simulink model "Project"  (R2024a)
settings: Solver=FixedStepDiscrete  StartTime=0.0  StopTime=10.0  FixedStep=1e-3  RelTol=1e-3
settings Model: Creator=User  LastModifiedBy=User
settings OptimizationCC: DefaultParameterBehavior=Inlined  EnhancedBackFolding=on  PassReuseOutputArgsAs=Individual arguments  ZeroExternalMemoryAtStartup=off  ZeroInternalMemoryAtStartup=off  OptimizeBlockOrder=speed  DifferentSizesBufferReuse=on  OptimizationCustomize=off  EfficientTunableParamExpr=on
settings DebuggingCC: ParameterTunabilityLossMsg=error
settings HardwareCC: ProdBitPerPointer=32  ProdBitPerSizeT=32  ProdBitPerPtrDiffT=32  ProdLargestAtomicFloat=None  ProdWordSize=32  ProdHWDeviceType=Atmel->AVR (32-bit)
settings SFSimCC: MATLABDynamicMemAlloc=off
settings RTWCC: Description=Embedded Coder  SystemTargetFile=ert.tlc  TemplateMakefile=ert_default_tmf
settings CodeAppCC: ForceParamTrailComments=on  IgnoreCustomStorageClasses=off  OperatorAnnotations=on  SimulinkDataObjDesc=on  SFDataObjDesc=on  InsertBlockDesc=on
settings ERTTargetCC: TargetLangStandard=C99 (ISO)  GenerateSampleERTMain=on  InlinedParameterPlacement=NonHierarchical  ERTCustomFileTemplate=example_file_process.tlc

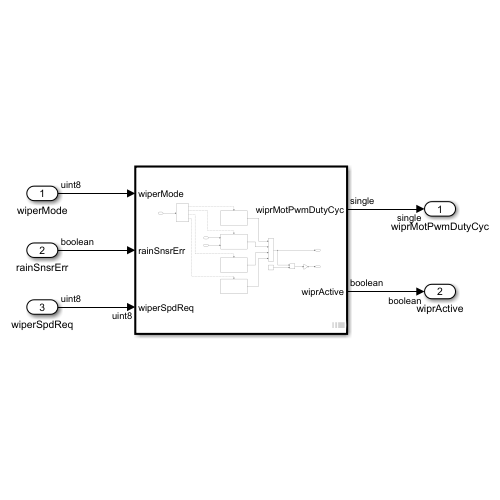
[thumbnail: Simulink's stored preview of the top-level diagram]
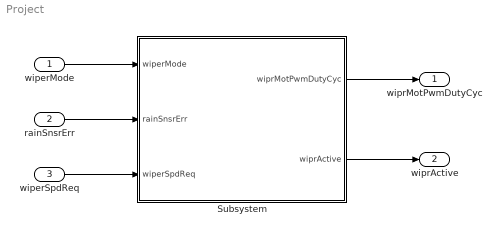
== system Project ==
  wiperMode : Inport  OutMin=0  OutMax=3  OutDataTypeStr=uint8
  rainSnsrErr : Inport  Port=2  OutMin=0  OutMax=1  OutDataTypeStr=boolean
  wiperSpdReq : Inport  Port=3  OutMin=0  OutMax=7  OutDataTypeStr=uint8
  Subsystem : Subsystem  TreatAsAtomicUnit=on
  wiprMotPwmDutyCyc : Outport  OutMin=0  OutMax=1  OutDataTypeStr=single
  wiprActive : Outport  Port=2  OutMin=0  OutMax=1  OutDataTypeStr=boolean
  wires:
  wiperSpdReq/1 -> Subsystem/3(wiperSpdReq)
  rainSnsrErr/1 -> Subsystem/2(rainSnsrErr)
  Subsystem/1(wiprMotPwmDutyCyc) -> wiprMotPwmDutyCyc/1
  Subsystem/2(wiprActive) -> wiprActive/1
  wiperMode/1 -> Subsystem/1(wiperMode)

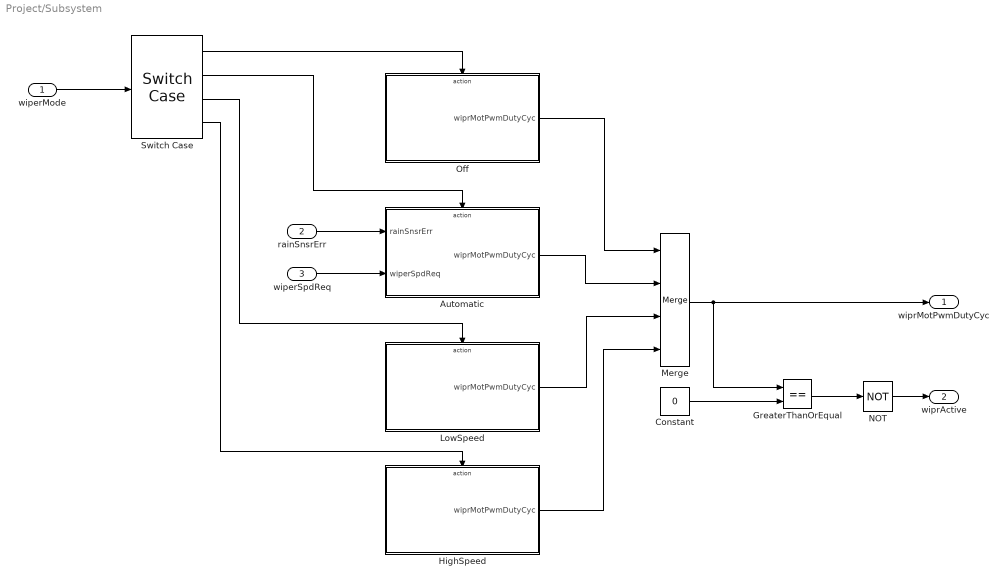
== system Project/Subsystem ==
  wiperMode : Inport
  rainSnsrErr : Inport  Port=2
  wiperSpdReq : Inport  Port=3  OutMin=0  OutMax=7  OutDataTypeStr=uint8
  Automatic : Subsystem  TreatAsAtomicUnit=on
  Constant : Constant  Value=0  OutDataTypeStr=single
  GreaterThanOrEqual : RelationalOperator  Operator===  OutDataTypeStr=boolean  RndMeth=Simplest  InputSameDT=off
  HighSpeed : Subsystem  TreatAsAtomicUnit=on
  LowSpeed : Subsystem  TreatAsAtomicUnit=on
  Merge : Merge  Inputs=4
  NOT : Logic  Operator=NOT  IconShape=distinctive  AllPortsSameDT=off  OutDataTypeStr=boolean
  Off : Subsystem  TreatAsAtomicUnit=on
  Switch Case : SwitchCase  CaseConditions={0,1,2,3}  ShowDefaultCase=off
  wiprMotPwmDutyCyc : Outport  OutMin=0  OutMax=1  OutDataTypeStr=single
  wiprActive : Outport  Port=2
  wires:
  wiperMode/1 -> Switch Case/1
  Switch Case/1 -> Off/Action
  Off/1(wiprMotPwmDutyCyc) -> Merge/1
  Merge/1 -> GreaterThanOrEqual/1, wiprMotPwmDutyCyc/1
  Switch Case/2 -> Automatic/Action
  rainSnsrErr/1 -> Automatic/1(rainSnsrErr)
  Automatic/1(wiprMotPwmDutyCyc) -> Merge/2
  wiperSpdReq/1 -> Automatic/2(wiperSpdReq)
  Switch Case/3 -> LowSpeed/Action
  Switch Case/4 -> HighSpeed/Action
  LowSpeed/1(wiprMotPwmDutyCyc) -> Merge/3
  HighSpeed/1(wiprMotPwmDutyCyc) -> Merge/4
  Constant/1 -> GreaterThanOrEqual/2
  GreaterThanOrEqual/1 -> NOT/1
  NOT/1 -> wiprActive/1

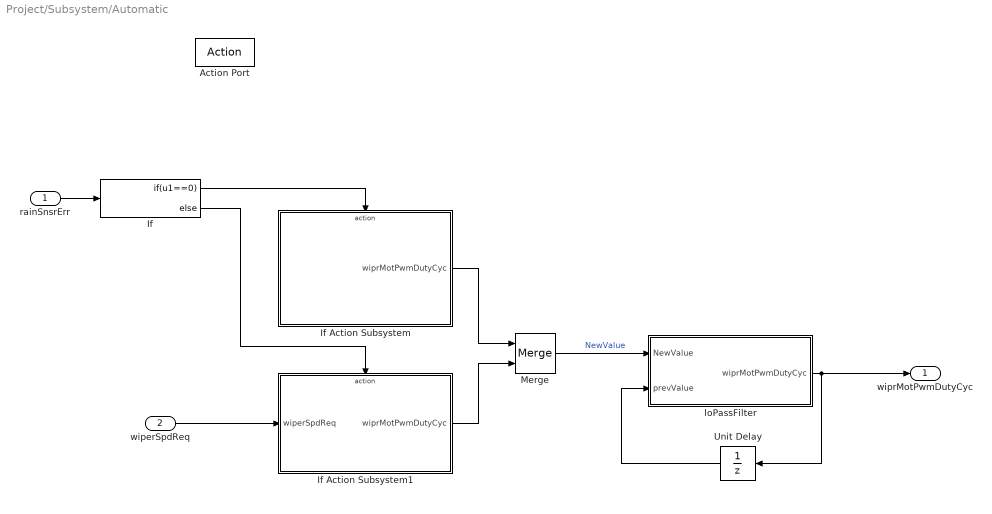
== system Project/Subsystem/Automatic ==
  rainSnsrErr : Inport
  wiperSpdReq : Inport  Port=2  OutMin=0  OutMax=7  OutDataTypeStr=uint8
  Action Port : ActionPort  ActionPortLabel=case [ 1 ]:
  If : If  IfExpression=u1==0
  If Action Subsystem : Subsystem  TreatAsAtomicUnit=on
  If Action Subsystem1 : Subsystem  TreatAsAtomicUnit=on
  Merge : Merge
  Unit Delay : UnitDelay  SampleTime=-1  HasFrameUpgradeWarning=on
  loPassFilter : Subsystem
  wiprMotPwmDutyCyc : Outport  OutMin=0  OutMax=1  OutDataTypeStr=single
  wires:
  rainSnsrErr/1 -> If/1
  If/1 -> If Action Subsystem/Action
  If Action Subsystem/1(wiprMotPwmDutyCyc) -> Merge/1
  Merge/1 -> loPassFilter/1(NewValue)  "NewValue"
  If/2 -> If Action Subsystem1/Action
  wiperSpdReq/1 -> If Action Subsystem1/1(wiperSpdReq)
  If Action Subsystem1/1(wiprMotPwmDutyCyc) -> Merge/2
  loPassFilter/1(wiprMotPwmDutyCyc) -> Unit Delay/1, wiprMotPwmDutyCyc/1
  Unit Delay/1 -> loPassFilter/2(prevValue)

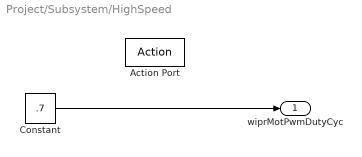
== system Project/Subsystem/HighSpeed ==
  Action Port : ActionPort  ActionPortLabel=case [ 3 ]:
  Constant : Constant  Value=.7  OutDataTypeStr=single
  wiprMotPwmDutyCyc : Outport  OutDataTypeStr=single
  wires:
  Constant/1 -> wiprMotPwmDutyCyc/1

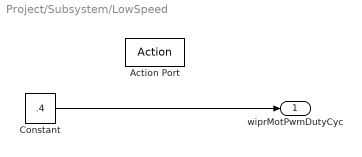
== system Project/Subsystem/LowSpeed ==
  Action Port : ActionPort  ActionPortLabel=case [ 2 ]:
  Constant : Constant  Value=.4  OutDataTypeStr=single
  wiprMotPwmDutyCyc : Outport  OutDataTypeStr=single
  wires:
  Constant/1 -> wiprMotPwmDutyCyc/1

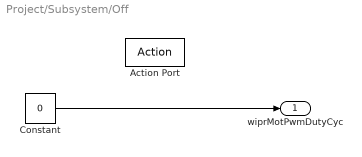
== system Project/Subsystem/Off ==
  Action Port : ActionPort  ActionPortLabel=case [ 0 ]:
  Constant : Constant  Value=0  OutDataTypeStr=single
  wiprMotPwmDutyCyc : Outport  OutDataTypeStr=single
  wires:
  Constant/1 -> wiprMotPwmDutyCyc/1

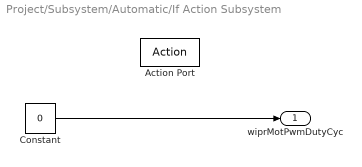
== system Project/Subsystem/Automatic/If Action Subsystem ==
  Action Port : ActionPort  ActionPortLabel=if(u1==0)
  Constant : Constant  Value=0  OutDataTypeStr=single
  wiprMotPwmDutyCyc : Outport  OutDataTypeStr=single
  wires:
  Constant/1 -> wiprMotPwmDutyCyc/1

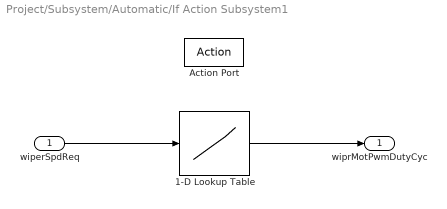
== system Project/Subsystem/Automatic/If Action Subsystem1 ==
  wiperSpdReq : Inport  OutMin=0  OutMax=7  OutDataTypeStr=uint8
  Action Port : ActionPort  ActionPortLabel=else
  1-D Lookup Table : Lookup_n-D  NumberOfTableDimensions=1  BreakpointsForDimension1=[0 1 2 3 4 5 6 7]  Table=[0 .4 .45 .5 .55 .6 .65 .7]  ExtrapMethod=Clip  InternalRulePriority=Speed  OutDataTypeStr=single  RndMeth=Simplest
  wiprMotPwmDutyCyc : Outport  OutMin=0  OutMax=1  OutDataTypeStr=single
  wires:
  1-D Lookup Table/1 -> wiprMotPwmDutyCyc/1
  wiperSpdReq/1 -> 1-D Lookup Table/1

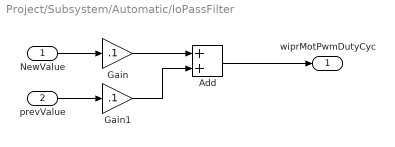
== system Project/Subsystem/Automatic/loPassFilter ==
  NewValue : Inport  OutDataTypeStr=single
  prevValue : Inport  Port=2  OutDataTypeStr=single
  Add : Sum
  Gain : Gain  Gain=.1
  Gain1 : Gain  Gain=.1
  wiprMotPwmDutyCyc : Outport  OutDataTypeStr=single
  wires:
  NewValue/1 -> Gain/1
  prevValue/1 -> Gain1/1
  Gain/1 -> Add/1
  Gain1/1 -> Add/2
  Add/1 -> wiprMotPwmDutyCyc/1
